simulink subsystem "Controls"  (R2024b)
settings: Solver=VariableStepAuto  StartTime=0.0  StopTime=10.0  RelTol=1e-3
undefined symbols (not defined in the file): D1, DiscIntNeverNeededParam, lag, Tctrl, test_alpha, Ts, Yg
libraries: powerlib_extras x74, simulink x10
(part 4 of 7)

== system Controls/Pole 1 Rectifier Control and Protection/Rectifier Controller/Voltage Error ==
  Vd_ref : Inport
  Vd_meas : Inport  Port=2
  Block : Inport  Port=3
  Id_err : Inport  Port=4
  Enable : EnablePort
  Constant1 : Constant  Value=0
  Constant2 : Constant  Value=0
  Constant3 : Constant  Value=Vd_marg
  Constant4 : Constant  Value=Id_marg
  Discrete 1st-Order Filter : powerlib_extras/Discrete  Control Blocks/Discrete 1st-Order Filter  FilterType=Highpass  Tc=0.01  Ts=dt  Initialize=off  Vac_Init=[0.8 -25 60]  Vdc_Init=-0.4  PlotResponse=off  param1=[1 500 0.1]
  MIN:eps MAX:inf : Saturate  UpperLimit=inf  LowerLimit=eps
  Math Function : Math  Operator=reciprocal  SignedPower=on
  Product1 : Product  Inputs=3  InputSameDT=on  SaturateOnIntegerOverflow=on  OutDataTypeStr=Inherit: Same as first input
  S6 : Subsystem  mask(Limiter with External Limits){}
      mask Display: disp('      Limiter\n')
  Sum3 : Sum  Inputs=+--  InputSameDT=on  SaturateOnIntegerOverflow=on  OutDataTypeStr=Inherit: Same as first input
  Switch2 : Switch  Threshold=0.5
  ERR_V : Outport
  wires:
  Sum3/1 -> Switch2/3
  Vd_ref/1 -> Sum3/1
  Vd_meas/1 -> Sum3/2
  Constant1/1 -> Switch2/1
  Block/1 -> Switch2/2
  Switch2/1 -> ERR_V/1  "ERR"
  Constant2/1 -> S6/3(MIN)
  S6/1("  ") -> Product1/3
  Math Function/1 -> Product1/2
  MIN:eps MAX:inf/1 -> Math Function/1
  Constant4/1 -> MIN:eps MAX:inf/1, S6/1(MAX)
  Product1/1 -> Discrete 1st-Order Filter/1
  Discrete 1st-Order Filter/1 -> Sum3/3  "dV"
  Id_err/1 -> S6/2(In)
  Constant3/1 -> Product1/1

== system Controls/Pole 1 Rectifier Control and Protection/Rectifier Controller/Voltage Regulator ==
  Max_i : Inport
  Min_i : Inport  Port=2
  ERR : Inport  Port=3
  Max_pi : Inport  Port=4
  Min_pi : Inport  Port=5
  Alpha_lin : Inport  Port=6
  Max_lin : Inport  Port=7
  Min_lin : Inport  Port=8
  Inv : Inport  Port=9
  Kp : Inport  Port=10
  Ki : Inport  Port=11
  Enable : EnablePort
  Voltage Regulator : Subsystem  mask(PI Regulator  With  External  Limits (Discrete)){Kp=Kp_V, Ki=Ki_V, IC_i=ICi_V, On_lin=on, pas=dt}
      mask prompts: Kp "Kp (deg/pu):"; Ki "Ki (deg/pu/s):"; IC_i "Integrator Initial Condition (deg):"; On_lin "Linearization  (On)"; pas "Sample time (s):"
      mask help: For the linearization it is important to specifie the mode of operation i.e. rectifier or inverter (negation of rectifier).
      mask Display: disp('PI Regulator\nWith external limits\n(Linearized Kp)\n(Discrete)\n\n')
  Alpha_ord : Outport
  wires:
  Kp/1 -> Voltage Regulator/10(Kp)
  Ki/1 -> Voltage Regulator/11(Ki)
  Voltage Regulator/1(Alpha_ord) -> Alpha_ord/1
  Max_i/1 -> Voltage Regulator/1(Max_i)
  Min_i/1 -> Voltage Regulator/2(Min_i)
  ERR/1 -> Voltage Regulator/3(ERR)
  Max_pi/1 -> Voltage Regulator/4(Max_pi)
  Min_pi/1 -> Voltage Regulator/5(Min_pi)
  Alpha_lin/1 -> Voltage Regulator/6(Alpha_lin)
  Max_lin/1 -> Voltage Regulator/7(Max_lin)
  Min_lin/1 -> Voltage Regulator/8(Min_lin)
  Inv/1 -> Voltage Regulator/9(Inv)

== system Controls/Pole 1 Rectifier Control and Protection/Rectifier Controller/alpha_init ==
  In1 : Inport  PortDimensions=1
  IC : InitialCondition  Value=min([ICi_V,ICi_I,ICi_G])
  Out1 : Outport
  wires:
  In1/1 -> IC/1
  IC/1 -> Out1/1

== system Controls/Pole 1 Rectifier Control and Protection/Rectifier Protections/DC Fault Protection (DCPROT) ==
  note: DC Fault Protection (only in Rectifier)
  VdL (pu) : Inport
  Deblocked : Inport  Port=2  OutDataTypeStr=boolean
  Lock : Inport  Port=3
  Enabled Subsystem : Subsystem  TreatAsAtomicUnit=on
  Forced_alpha : Outport
  wires:
  Enabled Subsystem/1(Forced_alpha) -> Forced_alpha/1
  Deblocked/1 -> Enabled Subsystem/2(Deblocked)
  Lock/1 -> Enabled Subsystem/3(Lock)
  VdL (pu)/1 -> Enabled Subsystem/1(VdL (pu))

== system Controls/Pole 1 Rectifier Control and Protection/Rectifier Protections/Informations ==
  note: The DC fault protection (DCPROT) and the Low AC voltage detection (LACVD) constitutes the
      | protectives functions at the rectifier. The DC fault protection detects a fault on the DC line and tries to
      | extinguish the fault current by ordering a Forced alpha operation during a fixed duration.
  note: DESCRIPTION
  note: Silvano Casoria (Hydro-Quebec)
  note: DC Protections - Rectifier
  note: The LACVD detects a low AC voltage condition on the rectifier commutation bus and sends a signal
      | (Lock) to the DCPROT in order to prevent the detection of a DC fault when the drop in the DC voltage is
      | due to a fault on the AC side. The LACVD at the inverter sends also a signal to lock the DCPROT for the
      | same reason.
  note: The  DCPROT detects a fault on the DC line and tries to extinguish the fault current by ordering a Forced
      | alpha operation for a fixed duration.

== system Controls/Pole 1 Rectifier Control and Protection/Rectifier Protections/Low AC Voltage Detection (LACVD) ==
  note: Low AC Voltage Detection
  Uac (pu) : Inport
  Enabled Subsystem : Subsystem  TreatAsAtomicUnit=on
  Low_AC_Voltage : Outport
  wires:
  Enabled Subsystem/1(Low_AC_Voltage) -> Low_AC_Voltage/1
  Uac (pu)/1 -> Enabled Subsystem/1(Uac (pu))

== system Controls/Pole 1 Rectifier Control and Protection/Rectifier Protections/Udio_6p ==
  note: Silvano Casoria
      | Power System Laboratory, IREQ
      | Hydro-Quebec
  note: Three-phase full-wave rectification
  Uabc (pu) : Inport
  MinMax : MinMax  Function=max  InputSameDT=on  SaturateOnIntegerOverflow=on
  MinMax1 : MinMax  InputSameDT=on  SaturateOnIntegerOverflow=on
  Sum : Sum  Inputs=+-  InputSameDT=on  SaturateOnIntegerOverflow=on  OutDataTypeStr=Inherit: Same as first input
  conversion pu ac->dc : Gain  Gain=pi/(3*sqrt(3))  SaturateOnIntegerOverflow=on  OutDataTypeStr=Inherit: Same as input  ParamDataTypeStr=Inherit: Same as input
  Udio_6p : Outport
  wires:
  MinMax1/1 -> Sum/2
  MinMax/1 -> Sum/1
  Uabc (pu)/1 -> MinMax/1, MinMax1/1
  Sum/1 -> conversion pu ac->dc/1
  conversion pu ac->dc/1 -> Udio_6p/1

== system Controls/Pole 2 Inverter Control and Protection/12-pulse Firing Control/PLL ==
  Vabc(pu) : Inport
  Constant : Constant  Value=2*pi/3
  Discrete 3-phase PLL : powerlib_extras/Discrete  Control Blocks/Discrete 3-phase PLL  Fmin=0.75 * PLL_f0  Par_Init="[PLL_ph  PLL_f0]"  ParK="[PLL_Kp  PLL_Ki]"  Ts=dt  AGC=off
  Sum : Sum  Inputs=|+-  SaturateOnIntegerOverflow=on
  Sum1 : Sum  Inputs=|++  SaturateOnIntegerOverflow=on
  Terminator : Terminator
  Trigonometric Function : Trigonometry
  Trigonometric Function1 : Trigonometry
  Trigonometric Function2 : Trigonometry
  Va : Outport
  Vb : Outport  Port=2
  Vc : Outport  Port=3
  Freq : Outport  Port=4
  wires:
  Discrete 3-phase PLL/3 -> Terminator/1
  Trigonometric Function2/1 -> Vc/1
  Trigonometric Function1/1 -> Vb/1
  Trigonometric Function/1 -> Va/1
  Sum1/1 -> Trigonometric Function2/1
  Constant/1 -> Sum/2, Sum1/2
  Sum/1 -> Trigonometric Function1/1
  Discrete 3-phase PLL/2 -> Sum1/1, Sum/1, Trigonometric Function/1
  Vabc(pu)/1 -> Discrete 3-phase PLL/1
  Discrete 3-phase PLL/1 -> Freq/1

== system Controls/Pole 2 Inverter Control and Protection/Inverter Current //Voltage//Gamma Controller /Alpha Control ==
  Forced_alpha : Inport
  D_alpha : Inport  Port=2
  Constant1 : Constant  Value=alpha_min
  Constant2 : Constant  Value=alpha_max
  Constant3 : Constant  Value=test_alpha
  Data Type Conversion : DataTypeConversion  OutDataTypeStr=boolean
  Logical Operator : Logic  Operator=OR
  "Rate Limiter " : RateLimiter  RisingSlewLimit=PRate_fix  FallingSlewLimit=NRate_fix  SampleTimeMode=inherited
  "Rate Limiter   " : RateLimiter  RisingSlewLimit=PRate_fix  FallingSlewLimit=NRate_fix  SampleTimeMode=inherited
  Sum : Sum  Inputs=-+  InputSameDT=on  SaturateOnIntegerOverflow=on  OutDataTypeStr=Inherit: Same as first input
  Switch : Switch  Threshold=0.5
  Switch1 : Switch  Threshold=0.5
  fixed alpha (deg) : Constant  Value=alpha_fix
  Max_i : Outport
  Min_i : Outport  Port=2
  wires:
  Data Type Conversion/1 -> Logical Operator/2
  Forced_alpha/1 -> Data Type Conversion/1
  fixed alpha (deg)/1 -> Switch1/1, Switch/1
  Switch1/1 -> "Rate Limiter   "/1
  Switch/1 -> "Rate Limiter "/1
  Constant1/1 -> Switch1/3
  Logical Operator/1 -> Switch1/2, Switch/2
  Constant3/1 -> Logical Operator/1
  Constant2/1 -> Sum/2
  Sum/1 -> Switch/3
  D_alpha/1 -> Sum/1
  "Rate Limiter "/1 -> Max_i/1
  "Rate Limiter   "/1 -> Min_i/1

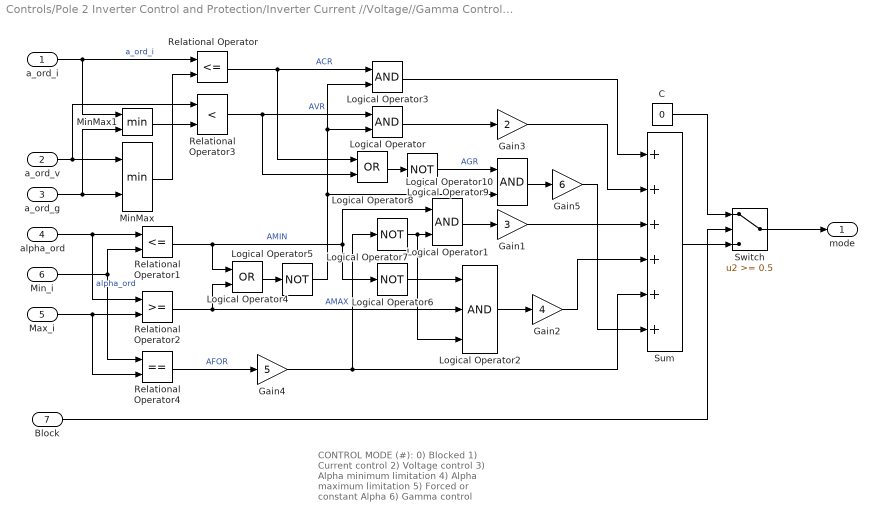
== system Controls/Pole 2 Inverter Control and Protection/Inverter Current //Voltage//Gamma Controller /Control Mode  ==
  note: CONTROL MODE (#):
      |
      | 0) Blocked
      | 1) Current control
      | 2) Voltage control
      | 3) Alpha minimum limitation
      | 4) Alpha maximum limitation
      | 5) Forced or constant Alpha
      | 6) Gamma control
  "a_ord_i " : Inport
  a_ord_v : Inport  Port=2
  a_ord_g : Inport  Port=3
  alpha_ord : Inport  Port=4
  Max_i : Inport  Port=5
  Min_i : Inport  Port=6
  Block : Inport  Port=7
  C : Constant  Value=0
  Gain1 : Gain  Gain=3  SaturateOnIntegerOverflow=on  OutDataTypeStr=Inherit: Same as input  ParamDataTypeStr=Inherit: Same as input
  Gain2 : Gain  Gain=4  SaturateOnIntegerOverflow=on  OutDataTypeStr=Inherit: Same as input  ParamDataTypeStr=Inherit: Same as input
  Gain3 : Gain  Gain=2  SaturateOnIntegerOverflow=on  OutDataTypeStr=Inherit: Same as input  ParamDataTypeStr=Inherit: Same as input
  Gain4 : Gain  Gain=5  SaturateOnIntegerOverflow=on  OutDataTypeStr=Inherit: Same as input  ParamDataTypeStr=Inherit: Same as input
  Gain5 : Gain  Gain=6  SaturateOnIntegerOverflow=on  OutDataTypeStr=Inherit: Same as input  ParamDataTypeStr=Inherit: Same as input
  Logical Operator{,1,3,10} (4 alike) : Logic
  Logical Operator2 : Logic  Inputs=3
  Logical Operator4 : Logic  Operator=OR
  Logical Operator{5..7,9} (4 alike) : Logic  Operator=NOT
  Logical Operator8 : Logic  Operator=OR
  MinMax : MinMax  Inputs=2  InputSameDT=on  SaturateOnIntegerOverflow=on
  MinMax1 : MinMax  Inputs=2  InputSameDT=on  SaturateOnIntegerOverflow=on
  Relational Operator : RelationalOperator  Operator=<=
  Relational Operator1 : RelationalOperator  Operator=<=
  Relational Operator2 : RelationalOperator
  Relational Operator3 : RelationalOperator  Operator=<
  Relational Operator4 : RelationalOperator  Operator===
  Sum : Sum  Inputs=++++++  InputSameDT=on  SaturateOnIntegerOverflow=on  OutDataTypeStr=Inherit: Same as first input
  Switch : Switch  Threshold=0.5
  mode : Outport
  wires:
  Logical Operator10/1 -> Gain5/1
  Logical Operator9/1 -> Logical Operator10/1  "AGR"
  MinMax1/1 -> Relational Operator3/2
  Gain5/1 -> Sum/6
  Logical Operator8/1 -> Logical Operator9/1
  MinMax/1 -> Relational Operator/2
  a_ord_g/1 -> MinMax1/2, MinMax/2
  a_ord_v/1 -> Relational Operator3/1, MinMax/1
  C/1 -> Switch/1
  Sum/1 -> Switch/3
  Switch/1 -> mode/1
  Block/1 -> Switch/2
  "a_ord_i "/1 -> MinMax1/1, Relational Operator/1  "a_ord_i"
  Relational Operator/1 -> Logical Operator8/1, Logical Operator3/1  "ACR"
  Logical Operator3/1 -> Sum/1
  Gain3/1 -> Sum/2
  Relational Operator3/1 -> Logical Operator8/2, Logical Operator/1  "AVR"
  Logical Operator/1 -> Gain3/1
  alpha_ord/1 -> Relational Operator1/1, Relational Operator2/1  "alpha_ord"
  Relational Operator1/1 -> Logical Operator4/1, Logical Operator6/1, Logical Operator1/1  "AMIN"
  Logical Operator4/1 -> Logical Operator5/1
  Relational Operator2/1 -> Logical Operator4/2, Logical Operator2/2  "AMAX"
  Logical Operator6/1 -> Logical Operator2/1
  Logical Operator2/1 -> Gain2/1
  Gain1/1 -> Sum/3
  Gain2/1 -> Sum/4
  Min_i/1 -> Relational Operator1/2, Relational Operator4/1
  Max_i/1 -> Relational Operator2/2, Relational Operator4/2
  Relational Operator4/1 -> Gain4/1  "AFOR"
  Logical Operator1/1 -> Gain1/1
  Gain4/1 -> Sum/5, Logical Operator7/1
  Logical Operator7/1 -> Logical Operator1/2, Logical Operator2/3
  Logical Operator5/1 -> Logical Operator10/2, Logical Operator/2, Logical Operator3/2

== system Controls/Pole 2 Inverter Control and Protection/Inverter Current //Voltage//Gamma Controller /Current Regulator ==
  note: PI Regulator With external limits (Linearized Kp) (Discrete)
  Max_i : Inport
  Min_i : Inport  Port=2
  ERR : Inport  Port=3
  Max_pi : Inport  Port=4
  Min_pi : Inport  Port=5
  Alpha_lin : Inport  Port=6
  Max_lin : Inport  Port=7
  Min_lin : Inport  Port=8
  Inv : Inport  Port=9
  Kp : Inport  Port=10
  Ki : Inport  Port=11
  Ground : Ground
  KI (deg per pu per s) : Gain  Gain=Ki  SaturateOnIntegerOverflow=on  OutDataTypeStr=Inherit: Same as input  ParamDataTypeStr=Inherit: Same as input
  Kp (deg per pu) : Constant  Value=Kp
  Kp Linearisation : Subsystem
  Prod : Product  InputSameDT=on  SaturateOnIntegerOverflow=on  OutDataTypeStr=Inherit: Same as first input
  Prod1 : Product  InputSameDT=on  SaturateOnIntegerOverflow=on  OutDataTypeStr=Inherit: Same as first input
  S16 : Subsystem  mask(Integrator  With  External  Dynamic  Limits (Discrete)){k=1, ic=IC_i, dt=dt}
      mask prompts: k "Gain:"; ic "Initial Condition:"; dt "Sample time: (s)"
      mask Display: disp('Integrator\nwith\nExternal Limits\nGain & Reset & Hold\n(Discrete)')
  S6 : Subsystem  mask(Limiter with External Limits){}
      mask Display: disp('      Limiter\n')
  Sum : Sum  InputSameDT=on  SaturateOnIntegerOverflow=on  OutDataTypeStr=Inherit: Same as first input
  Alpha_ord : Outport  InitialOutput=0
  wires:
  Prod1/1 -> S16/3(In)
  Ki/1 -> Prod1/2
  Kp/1 -> Kp Linearisation/2(Kp)
  Prod/1 -> Sum/1
  Min_lin/1 -> Kp Linearisation/4(Min_lin)
  Max_lin/1 -> Kp Linearisation/5(Max_lin)
  Inv/1 -> Kp Linearisation/3(Inv)
  Ground/1 -> S16/6(Reset Value), S16/5(Hold), S16/4(Reset)
  ERR/1 -> Prod1/1, Prod/2, KI (deg per pu per s)/1
  S16/1(Out) -> Sum/2
  Min_pi/1 -> S6/3(MIN)
  Max_pi/1 -> S6/1(MAX)
  Sum/1 -> S6/2(In)
  Min_i/1 -> S16/2(Min)
  Max_i/1 -> S16/1(Max)
  Kp Linearisation/1(Kp_lin) -> Prod/1
  S6/1("  ") -> Alpha_ord/1
  Alpha_lin/1 -> Kp Linearisation/1(Alpha_lin)

== system Controls/Pole 2 Inverter Control and Protection/Inverter Current //Voltage//Gamma Controller /Gamma Error ==
  G_ref : Inport
  G_meas : Inport  Port=2
  Block : Inport  Port=3
  Id_err : Inport  Port=4
  Enable : EnablePort
  Constant1 : Constant  Value=0
  Constant2 : Constant  Value=0
  Constant3 : Constant  Value=G_marg
  Constant4 : Constant  Value=Id_marg
  Discrete 1st-Order Filter : powerlib_extras/Discrete  Control Blocks/Discrete 1st-Order Filter  FilterType=Highpass  Tc=0.01  Ts=dt  Initialize=off  Vac_Init=[0.8 -25 60]  Vdc_Init=-0.4  PlotResponse=off  param1=[1 500 0.1]
  MIN:eps MAX:inf : Saturate  UpperLimit=inf  LowerLimit=eps
  Math Function : Math  Operator=reciprocal  SignedPower=on
  Product1 : Product  Inputs=3  InputSameDT=on  SaturateOnIntegerOverflow=on  OutDataTypeStr=Inherit: Same as first input
  S6 : Subsystem  mask(Limiter with External Limits){}
      mask Display: disp('      Limiter\n')
  Sum3 : Sum  Inputs=-+-  InputSameDT=on  SaturateOnIntegerOverflow=on  OutDataTypeStr=Inherit: Same as first input
  Switch2 : Switch  Threshold=0.5
  ERR_G : Outport
  wires:
  Constant3/1 -> Product1/1
  Id_err/1 -> S6/2(In)
  Discrete 1st-Order Filter/1 -> Sum3/3  "dG"
  Product1/1 -> Discrete 1st-Order Filter/1
  Constant4/1 -> S6/1(MAX), MIN:eps MAX:inf/1
  MIN:eps MAX:inf/1 -> Math Function/1
  Math Function/1 -> Product1/2
  S6/1("  ") -> Product1/3
  Constant2/1 -> S6/3(MIN)
  Switch2/1 -> ERR_G/1  "ERR"
  Block/1 -> Switch2/2
  Constant1/1 -> Switch2/1
  G_meas/1 -> Sum3/2
  G_ref/1 -> Sum3/1
  Sum3/1 -> Switch2/3

== system Controls/Pole 2 Inverter Control and Protection/Inverter Current //Voltage//Gamma Controller /Gamma Regulator ==
  Max_i : Inport
  Min_i : Inport  Port=2
  ERR : Inport  Port=3
  Max_pi : Inport  Port=4
  Min_pi : Inport  Port=5
  Alpha_lin : Inport  Port=6
  Max_lin : Inport  Port=7
  Min_lin : Inport  Port=8
  Inv : Inport  Port=9
  Kp : Inport  Port=10
  Ki : Inport  Port=11
  Enable : EnablePort
  Gamma Regulator : Subsystem  mask(PI Regulator  With  External  Limits (Discrete)){Kp=Kp_G, Ki=Ki_G, IC_i=ICi_G, On_lin=on, pas=dt}
      mask prompts: Kp "Kp (deg/pu):"; Ki "Ki (deg/pu/s):"; IC_i "Integrator Initial Condition (deg):"; On_lin "Linearization  (On)"; pas "Sample time (s):"
      mask help: For the linearization it is important to specifie the mode of operation i.e. rectifier or inverter (negation of rectifier).
      mask Display: disp('PI Regulator\nWith external limits\n(Linearized Kp)\n(Discrete)\n\n')
  Alpha_ord : Outport
  wires:
  Ki/1 -> Gamma Regulator/11(Ki)
  Kp/1 -> Gamma Regulator/10(Kp)
  Inv/1 -> Gamma Regulator/9(Inv)
  Min_lin/1 -> Gamma Regulator/8(Min_lin)
  Max_lin/1 -> Gamma Regulator/7(Max_lin)
  Alpha_lin/1 -> Gamma Regulator/6(Alpha_lin)
  Min_pi/1 -> Gamma Regulator/5(Min_pi)
  Max_pi/1 -> Gamma Regulator/4(Max_pi)
  ERR/1 -> Gamma Regulator/3(ERR)
  Min_i/1 -> Gamma Regulator/2(Min_i)
  Max_i/1 -> Gamma Regulator/1(Max_i)
  Gamma Regulator/1(Alpha_ord) -> Alpha_ord/1

== system Controls/Pole 2 Inverter Control and Protection/Inverter Current //Voltage//Gamma Controller /Voltage Dependant Current Order Limiter ==
  note: Voltage Dependant Current Order Limiter (VDCOL) (Discrete)
  Id_ref (pu) : Inport
  Vd (pu) : Inport  Port=2
  Constant : Constant  Value=Id_min
  Constant1 : Constant  Value=Vd_min
  Constant2 : Constant  Value=Vd_seuil
  Constant3 : Constant
  Constant4 : Constant
  Constant5 : Constant  Value=Tu
  Logical Operator : Logic  Operator=NOT
  Math Function : Math  Operator=reciprocal  SignedPower=on
  Max = 10 Min=Id_min_abs : Saturate  UpperLimit=10  LowerLimit=Id_min_abs
  MinMax2 : MinMax  Function=max  Inputs=2  InputSameDT=on  SaturateOnIntegerOverflow=on
  MinMax3 : MinMax  Inputs=2  InputSameDT=on  SaturateOnIntegerOverflow=on
  PB_R : Subsystem  mask(Low Pass Filter With Reset (discrete: Zoh method, Forward Euler)){ic=1, dt=pas}
      mask prompts: ic "Initial condition:"; dt "Sample time (s)"
      mask help:
      | The output will be reset to the input value (Time constant = 0)  during the input (2) is True. The Time constant (T) is defined by
      | input (3).
      mask Display:
      | plot(0,0,100,100,[90,80,70,60,50,40,29,20,10],[60,55,52,55,60,65,67,65,60],[89,80,71,60,50,40,30,20,10],[40,35,32,35,40,45,47,45,40],[56,44],[70,50]);
      | disp('\n\nD')
  Product : Product  InputSameDT=on  SaturateOnIntegerOverflow=on
  Product1 : Product  InputSameDT=on  SaturateOnIntegerOverflow=on
  Product2 : Product  InputSameDT=on  SaturateOnIntegerOverflow=on  OutDataTypeStr=Inherit: Same as first input
  Product3 : Product  InputSameDT=on  SaturateOnIntegerOverflow=on  OutDataTypeStr=Inherit: Same as first input
  Product4 : Product  InputSameDT=on  SaturateOnIntegerOverflow=on  OutDataTypeStr=Inherit: Same as first input
  Relational Operator : RelationalOperator
  Sum : Sum  Inputs=+-  InputSameDT=on  SaturateOnIntegerOverflow=on  OutDataTypeStr=Inherit: Same as first input
  Sum1 : Sum  Inputs=+-  InputSameDT=on  SaturateOnIntegerOverflow=on  OutDataTypeStr=Inherit: Same as first input
  Sum2 : Sum  Inputs=+-  InputSameDT=on  SaturateOnIntegerOverflow=on  OutDataTypeStr=Inherit: Same as first input
  Sum3 : Sum  InputSameDT=on  SaturateOnIntegerOverflow=on  OutDataTypeStr=Inherit: Same as first input
  Unit Delay : UnitDelay  SampleTime=pas  HasFrameUpgradeWarning=on
  Id_ref_lim : Outport  InitialOutput=0
  Vd_filt : Outport  Port=2  InitialOutput=0
  wires:
  Logical Operator/1 -> PB_R/2(Reset)
  Unit Delay/1 -> Logical Operator/1
  Vd (pu)/1 -> Relational Operator/1, PB_R/1("In ")
  PB_R/1(Out) -> Relational Operator/2, Vd_filt/1, Product2/2
  Constant5/1 -> PB_R/3(T)
  Constant3/1 -> Sum/1
  Constant1/1 -> Sum1/2
  Sum1/1 -> Math Function/1
  Sum/1 -> Product/1
  Math Function/1 -> Product/2
  Constant4/1 -> Sum2/1
  Sum2/1 -> Sum3/1  "B"
  Product2/1 -> Sum3/2
  Sum3/1 -> Product1/2
  Constant/1 -> Sum/2, Product4/1
  Product4/1 -> Max = 10 Min=Id_min_abs/1  "min"
  Id_ref (pu)/1 -> Product1/1, MinMax3/1, Product4/2
  MinMax3/1 -> Id_ref_lim/1
  Product3/1 -> Sum2/2
  Product/1 -> Product2/1, Product3/2  "A"
  Constant2/1 -> Sum1/1, Product3/1
  Product1/1 -> MinMax2/1  "Idref_lim"
  MinMax2/1 -> MinMax3/2
  Max = 10 Min=Id_min_abs/1 -> MinMax2/2
  Relational Operator/1 -> Unit Delay/1

== system Controls/Pole 2 Inverter Control and Protection/Inverter Current //Voltage//Gamma Controller /Voltage Error ==
  Vd_ref : Inport
  Vd_meas : Inport  Port=2
  Block : Inport  Port=3
  Id_err : Inport  Port=4
  Enable : EnablePort
  Constant1 : Constant  Value=0
  Constant2 : Constant  Value=0
  Constant3 : Constant  Value=Vd_marg
  Constant4 : Constant  Value=Id_marg
  Discrete 1st-Order Filter : powerlib_extras/Discrete  Control Blocks/Discrete 1st-Order Filter  FilterType=Highpass  Tc=0.01  Ts=dt  Initialize=off  Vac_Init=[0.8 -25 60]  Vdc_Init=-0.4  PlotResponse=off  param1=[1 500 0.1]
  MIN:eps MAX:inf : Saturate  UpperLimit=inf  LowerLimit=eps
  Math Function : Math  Operator=reciprocal  SignedPower=on
  Product1 : Product  Inputs=3  InputSameDT=on  SaturateOnIntegerOverflow=on  OutDataTypeStr=Inherit: Same as first input
  S6 : Subsystem  mask(Limiter with External Limits){}
      mask Display: disp('      Limiter\n')
  Sum3 : Sum  Inputs=+--  InputSameDT=on  SaturateOnIntegerOverflow=on  OutDataTypeStr=Inherit: Same as first input
  Switch2 : Switch  Threshold=0.5
  ERR_V : Outport
  wires:
  Sum3/1 -> Switch2/3
  Vd_ref/1 -> Sum3/1
  Vd_meas/1 -> Sum3/2
  Constant1/1 -> Switch2/1
  Block/1 -> Switch2/2
  Switch2/1 -> ERR_V/1  "ERR"
  Constant2/1 -> S6/3(MIN)
  S6/1("  ") -> Product1/3
  Math Function/1 -> Product1/2
  MIN:eps MAX:inf/1 -> Math Function/1
  Constant4/1 -> MIN:eps MAX:inf/1, S6/1(MAX)
  Product1/1 -> Discrete 1st-Order Filter/1
  Discrete 1st-Order Filter/1 -> Sum3/3  "dV"
  Id_err/1 -> S6/2(In)
  Constant3/1 -> Product1/1

== system Controls/Pole 2 Inverter Control and Protection/Inverter Current //Voltage//Gamma Controller /Voltage Regulator ==
  Max_i : Inport
  Min_i : Inport  Port=2
  ERR : Inport  Port=3
  Max_pi : Inport  Port=4
  Min_pi : Inport  Port=5
  Alpha_lin : Inport  Port=6
  Max_lin : Inport  Port=7
  Min_lin : Inport  Port=8
  Inv : Inport  Port=9
  Kp : Inport  Port=10
  Ki : Inport  Port=11
  Enable : EnablePort
  Voltage Regulator : Subsystem  mask(PI Regulator  With  External  Limits (Discrete)){Kp=Kp_V, Ki=Ki_V, IC_i=ICi_V, On_lin=on, pas=dt}
      mask prompts: Kp "Kp (deg/pu):"; Ki "Ki (deg/pu/s):"; IC_i "Integrator Initial Condition (deg):"; On_lin "Linearization  (On)"; pas "Sample time (s):"
      mask help: For the linearization it is important to specifie the mode of operation i.e. rectifier or inverter (negation of rectifier).
      mask Display: disp('PI Regulator\nWith external limits\n(Linearized Kp)\n(Discrete)\n\n')
  Alpha_ord : Outport
  wires:
  Ki/1 -> Voltage Regulator/11(Ki)
  Kp/1 -> Voltage Regulator/10(Kp)
  Voltage Regulator/1(Alpha_ord) -> Alpha_ord/1
  Max_i/1 -> Voltage Regulator/1(Max_i)
  Min_i/1 -> Voltage Regulator/2(Min_i)
  ERR/1 -> Voltage Regulator/3(ERR)
  Max_pi/1 -> Voltage Regulator/4(Max_pi)
  Min_pi/1 -> Voltage Regulator/5(Min_pi)
  Alpha_lin/1 -> Voltage Regulator/6(Alpha_lin)
  Max_lin/1 -> Voltage Regulator/7(Max_lin)
  Min_lin/1 -> Voltage Regulator/8(Min_lin)
  Inv/1 -> Voltage Regulator/9(Inv)

== system Controls/Pole 2 Inverter Control and Protection/Inverter Current //Voltage//Gamma Controller /alpha_init ==
  In1 : Inport  PortDimensions=1
  IC : InitialCondition  Value=min([ICi_V,ICi_I,ICi_G])
  Out1 : Outport
  wires:
  In1/1 -> IC/1
  IC/1 -> Out1/1

== system Controls/Pole 2 Inverter Control and Protection/Inverter Protections/Commutation Failure Prevention Control (CFPREV) ==
  note: Commutation failure Prevention Control Module (CFPREV)
  Uabc (pu) : Inport
  C : Constant  Value=STATE
  Enabled Subsystem : Subsystem  TreatAsAtomicUnit=on
  AMIN_CFPREV (deg) : Outport
  wires:
  Enabled Subsystem/1(AMIN_CFPREV (deg)) -> AMIN_CFPREV (deg)/1
  Uabc (pu)/1 -> Enabled Subsystem/1(Uabc (pu))
  C/1 -> Enabled Subsystem/Enable

== system Controls/Pole 2 Inverter Control and Protection/Inverter Protections/Informations ==
  note: NOTE 1: Result of a failure of the incoming valve to take over the direct current before the commutating voltage reverses its polarity.
  note: DC Protections - Inverter
  note: DESCRIPTION
  note: The LACVD detects a low AC voltage condition on the inverter commutation bus and sends a signal
      | (Lock) to the DCPROT (in the rectifier) in order to prevent the detection of a DC fault when the drop in
      | the DC voltage is due to a fault on the AC side. The LACVD at the irectifier sends also a signal to
      | lock the DCPROT for the same reason.
  note: The Commutation failure prevention control (CFPREV) and the Low AC voltage detection (LACVD)
      | constitutes the protective functions at the rinverter.
  note: The CFPREV  mitigates commutation failures due to AC voltage dips. After a fault detection (three-phase or
      | one-phase) an angle value (AMIN_CFPREV) is sent to the converter control in order to be deducted from the
      | maximum delay angle limit (alpha_max). In practice, the commutation margin is consequently enlarged
      | reducing therefore the risk of commutation failures (note 1).

== system Controls/Pole 2 Inverter Control and Protection/Inverter Protections/Low AC Voltage Detection (LACVD) ==
  note: Low AC Voltage Detection
  Uac (pu) : Inport
  Enabled Subsystem : Subsystem  TreatAsAtomicUnit=on
  Low_AC_Voltage : Outport
  wires:
  Enabled Subsystem/1(Low_AC_Voltage) -> Low_AC_Voltage/1
  Uac (pu)/1 -> Enabled Subsystem/1(Uac (pu))

== system Controls/Pole 2 Inverter Control and Protection/Inverter Protections/Udio_6p ==
  note: Three-phase full-wave rectification
  note: Silvano Casoria
      | Power System Laboratory, IREQ
      | Hydro-Quebec
  Uabc (pu) : Inport
  MinMax : MinMax  Function=max  InputSameDT=on  SaturateOnIntegerOverflow=on
  MinMax1 : MinMax  InputSameDT=on  SaturateOnIntegerOverflow=on
  Sum : Sum  Inputs=+-  InputSameDT=on  SaturateOnIntegerOverflow=on  OutDataTypeStr=Inherit: Same as first input
  conversion pu ac->dc : Gain  Gain=pi/(3*sqrt(3))  SaturateOnIntegerOverflow=on  OutDataTypeStr=Inherit: Same as input  ParamDataTypeStr=Inherit: Same as input
  Udio_6p : Outport
  wires:
  conversion pu ac->dc/1 -> Udio_6p/1
  Sum/1 -> conversion pu ac->dc/1
  Uabc (pu)/1 -> MinMax1/1, MinMax/1
  MinMax/1 -> Sum/1
  MinMax1/1 -> Sum/2

== system Controls/Pole 2 Rectifier Control and Protection/12-pulse Firing Control/PLL ==
  Vabc(pu) : Inport
  Constant : Constant  Value=2*pi/3
  Discrete 3-phase PLL : powerlib_extras/Discrete  Control Blocks/Discrete 3-phase PLL  Fmin=0.75 * PLL_f0  Par_Init="[PLL_ph  PLL_f0]"  ParK="[PLL_Kp  PLL_Ki]"  Ts=dt  AGC=off
  Sum : Sum  Inputs=|+-  SaturateOnIntegerOverflow=on
  Sum1 : Sum  Inputs=|++  SaturateOnIntegerOverflow=on
  Terminator : Terminator
  Trigonometric Function : Trigonometry
  Trigonometric Function1 : Trigonometry
  Trigonometric Function2 : Trigonometry
  Va : Outport
  Vb : Outport  Port=2
  Vc : Outport  Port=3
  Freq : Outport  Port=4
  wires:
  Discrete 3-phase PLL/3 -> Terminator/1
  Trigonometric Function2/1 -> Vc/1
  Trigonometric Function1/1 -> Vb/1
  Trigonometric Function/1 -> Va/1
  Sum1/1 -> Trigonometric Function2/1
  Constant/1 -> Sum/2, Sum1/2
  Sum/1 -> Trigonometric Function1/1
  Discrete 3-phase PLL/2 -> Sum1/1, Sum/1, Trigonometric Function/1
  Vabc(pu)/1 -> Discrete 3-phase PLL/1
  Discrete 3-phase PLL/1 -> Freq/1

== system Controls/Pole 2 Rectifier Control and Protection/Rectifier Controller/Alpha Control ==
  Forced_alpha : Inport
  D_alpha : Inport  Port=2
  Constant1 : Constant  Value=alpha_min
  Constant2 : Constant  Value=alpha_max
  Constant3 : Constant  Value=test_alpha
  Data Type Conversion : DataTypeConversion  OutDataTypeStr=boolean
  Logical Operator : Logic  Operator=OR
  "Rate Limiter " : RateLimiter  RisingSlewLimit=PRate_fix  FallingSlewLimit=NRate_fix  SampleTimeMode=inherited
  "Rate Limiter   " : RateLimiter  RisingSlewLimit=PRate_fix  FallingSlewLimit=NRate_fix  SampleTimeMode=inherited
  Sum : Sum  Inputs=-+  InputSameDT=on  SaturateOnIntegerOverflow=on  OutDataTypeStr=Inherit: Same as first input
  Switch : Switch  Threshold=0.5
  Switch1 : Switch  Threshold=0.5
  fixed alpha (deg) : Constant  Value=alpha_fix
  Max_i : Outport
  Min_i : Outport  Port=2
  wires:
  Data Type Conversion/1 -> Logical Operator/2
  Forced_alpha/1 -> Data Type Conversion/1
  fixed alpha (deg)/1 -> Switch1/1, Switch/1
  Switch1/1 -> "Rate Limiter   "/1
  Switch/1 -> "Rate Limiter "/1
  Constant1/1 -> Switch1/3
  Logical Operator/1 -> Switch1/2, Switch/2
  Constant3/1 -> Logical Operator/1
  Constant2/1 -> Sum/2
  Sum/1 -> Switch/3
  D_alpha/1 -> Sum/1
  "Rate Limiter "/1 -> Max_i/1
  "Rate Limiter   "/1 -> Min_i/1

== system Controls/Pole 2 Rectifier Control and Protection/Rectifier Controller/Control Mode  ==
  note: CONTROL MODE (#):
      |
      | 0) Blocked
      | 1) Current control
      | 2) Voltage control
      | 3) Alpha minimum limitation
      | 4) Alpha maximum limitation
      | 5) Forced or constant Alpha
      | 6) Gamma control
  "a_ord_i " : Inport
  a_ord_v : Inport  Port=2
  a_ord_g : Inport  Port=3
  alpha_ord : Inport  Port=4
  Max_i : Inport  Port=5
  Min_i : Inport  Port=6
  Block : Inport  Port=7
  C : Constant  Value=0
  Gain1 : Gain  Gain=3  SaturateOnIntegerOverflow=on  OutDataTypeStr=Inherit: Same as input  ParamDataTypeStr=Inherit: Same as input
  Gain2 : Gain  Gain=4  SaturateOnIntegerOverflow=on  OutDataTypeStr=Inherit: Same as input  ParamDataTypeStr=Inherit: Same as input
  Gain3 : Gain  Gain=2  SaturateOnIntegerOverflow=on  OutDataTypeStr=Inherit: Same as input  ParamDataTypeStr=Inherit: Same as input
  Gain4 : Gain  Gain=5  SaturateOnIntegerOverflow=on  OutDataTypeStr=Inherit: Same as input  ParamDataTypeStr=Inherit: Same as input
  Gain5 : Gain  Gain=6  SaturateOnIntegerOverflow=on  OutDataTypeStr=Inherit: Same as input  ParamDataTypeStr=Inherit: Same as input
  Logical Operator{,1,3,10} (4 alike) : Logic
  Logical Operator2 : Logic  Inputs=3
  Logical Operator4 : Logic  Operator=OR
  Logical Operator{5..7,9} (4 alike) : Logic  Operator=NOT
  Logical Operator8 : Logic  Operator=OR
  MinMax : MinMax  Inputs=2  InputSameDT=on  SaturateOnIntegerOverflow=on
  MinMax1 : MinMax  Inputs=2  InputSameDT=on  SaturateOnIntegerOverflow=on
  Relational Operator : RelationalOperator  Operator=<=
  Relational Operator1 : RelationalOperator  Operator=<=
  Relational Operator2 : RelationalOperator
  Relational Operator3 : RelationalOperator  Operator=<
  Relational Operator4 : RelationalOperator  Operator===
  Sum : Sum  Inputs=++++++  InputSameDT=on  SaturateOnIntegerOverflow=on  OutDataTypeStr=Inherit: Same as first input
  Switch : Switch  Threshold=0.5
  mode : Outport
  wires:
  Logical Operator10/1 -> Gain5/1
  Logical Operator9/1 -> Logical Operator10/1  "AGR"
  MinMax1/1 -> Relational Operator3/2
  Gain5/1 -> Sum/6
  Logical Operator8/1 -> Logical Operator9/1
  MinMax/1 -> Relational Operator/2
  a_ord_g/1 -> MinMax1/2, MinMax/2
  a_ord_v/1 -> Relational Operator3/1, MinMax/1
  C/1 -> Switch/1
  Sum/1 -> Switch/3
  Switch/1 -> mode/1
  Block/1 -> Switch/2
  "a_ord_i "/1 -> MinMax1/1, Relational Operator/1  "a_ord_i"
  Relational Operator/1 -> Logical Operator8/1, Logical Operator3/1  "ACR"
  Logical Operator3/1 -> Sum/1
  Gain3/1 -> Sum/2
  Relational Operator3/1 -> Logical Operator8/2, Logical Operator/1  "AVR"
  Logical Operator/1 -> Gain3/1
  alpha_ord/1 -> Relational Operator1/1, Relational Operator2/1  "alpha_ord"
  Relational Operator1/1 -> Logical Operator4/1, Logical Operator6/1, Logical Operator1/1  "AMIN"
  Logical Operator4/1 -> Logical Operator5/1
  Relational Operator2/1 -> Logical Operator4/2, Logical Operator2/2  "AMAX"
  Logical Operator6/1 -> Logical Operator2/1
  Logical Operator2/1 -> Gain2/1
  Gain1/1 -> Sum/3
  Gain2/1 -> Sum/4
  Min_i/1 -> Relational Operator1/2, Relational Operator4/1
  Max_i/1 -> Relational Operator2/2, Relational Operator4/2
  Relational Operator4/1 -> Gain4/1  "AFOR"
  Logical Operator1/1 -> Gain1/1
  Gain4/1 -> Sum/5, Logical Operator7/1
  Logical Operator7/1 -> Logical Operator1/2, Logical Operator2/3
  Logical Operator5/1 -> Logical Operator10/2, Logical Operator/2, Logical Operator3/2

== system Controls/Pole 2 Rectifier Control and Protection/Rectifier Controller/Current Regulator ==
  note: PI Regulator With external limits (Linearized Kp) (Discrete)
  Max_i : Inport
  Min_i : Inport  Port=2
  ERR : Inport  Port=3
  Max_pi : Inport  Port=4
  Min_pi : Inport  Port=5
  Alpha_lin : Inport  Port=6
  Max_lin : Inport  Port=7
  Min_lin : Inport  Port=8
  Inv : Inport  Port=9
  Kp : Inport  Port=10
  Ki : Inport  Port=11
  Ground : Ground
  KI (deg per pu per s) : Gain  Gain=Ki  SaturateOnIntegerOverflow=on  OutDataTypeStr=Inherit: Same as input  ParamDataTypeStr=Inherit: Same as input
  Kp (deg per pu) : Constant  Value=Kp
  Kp Linearisation : Subsystem
  Prod : Product  InputSameDT=on  SaturateOnIntegerOverflow=on  OutDataTypeStr=Inherit: Same as first input
  Prod1 : Product  InputSameDT=on  SaturateOnIntegerOverflow=on  OutDataTypeStr=Inherit: Same as first input
  S16 : Subsystem  mask(Integrator  With  External  Dynamic  Limits (Discrete)){k=1, ic=IC_i, dt=dt}
      mask prompts: k "Gain:"; ic "Initial Condition:"; dt "Sample time: (s)"
      mask Display: disp('Integrator\nwith\nExternal Limits\nGain & Reset & Hold\n(Discrete)')
  S6 : Subsystem  mask(Limiter with External Limits){}
      mask Display: disp('      Limiter\n')
  Sum : Sum  InputSameDT=on  SaturateOnIntegerOverflow=on  OutDataTypeStr=Inherit: Same as first input
  Alpha_ord : Outport  InitialOutput=0
  wires:
  Prod1/1 -> S16/3(In)
  Ki/1 -> Prod1/2
  Kp/1 -> Kp Linearisation/2(Kp)
  Prod/1 -> Sum/1
  Min_lin/1 -> Kp Linearisation/4(Min_lin)
  Max_lin/1 -> Kp Linearisation/5(Max_lin)
  Inv/1 -> Kp Linearisation/3(Inv)
  Ground/1 -> S16/6(Reset Value), S16/5(Hold), S16/4(Reset)
  ERR/1 -> Prod1/1, Prod/2, KI (deg per pu per s)/1
  S16/1(Out) -> Sum/2
  Min_pi/1 -> S6/3(MIN)
  Max_pi/1 -> S6/1(MAX)
  Sum/1 -> S6/2(In)
  Min_i/1 -> S16/2(Min)
  Max_i/1 -> S16/1(Max)
  Kp Linearisation/1(Kp_lin) -> Prod/1
  S6/1("  ") -> Alpha_ord/1
  Alpha_lin/1 -> Kp Linearisation/1(Alpha_lin)

== system Controls/Pole 2 Rectifier Control and Protection/Rectifier Controller/Gamma Error ==
  G_ref : Inport
  G_meas : Inport  Port=2
  Block : Inport  Port=3
  Id_err : Inport  Port=4
  Enable : EnablePort
  Constant1 : Constant  Value=0
  Constant2 : Constant  Value=0
  Constant3 : Constant  Value=G_marg
  Constant4 : Constant  Value=Id_marg
  Discrete 1st-Order Filter : powerlib_extras/Discrete  Control Blocks/Discrete 1st-Order Filter  FilterType=Highpass  Tc=0.01  Ts=dt  Initialize=off  Vac_Init=[0.8 -25 60]  Vdc_Init=-0.4  PlotResponse=off  param1=[1 500 0.1]
  MIN:eps MAX:inf : Saturate  UpperLimit=inf  LowerLimit=eps
  Math Function : Math  Operator=reciprocal  SignedPower=on
  Product1 : Product  Inputs=3  InputSameDT=on  SaturateOnIntegerOverflow=on  OutDataTypeStr=Inherit: Same as first input
  S6 : Subsystem  mask(Limiter with External Limits){}
      mask Display: disp('      Limiter\n')
  Sum3 : Sum  Inputs=-+-  InputSameDT=on  SaturateOnIntegerOverflow=on  OutDataTypeStr=Inherit: Same as first input
  Switch2 : Switch  Threshold=0.5
  ERR_G : Outport
  wires:
  Constant3/1 -> Product1/1
  Id_err/1 -> S6/2(In)
  Discrete 1st-Order Filter/1 -> Sum3/3  "dG"
  Product1/1 -> Discrete 1st-Order Filter/1
  Constant4/1 -> S6/1(MAX), MIN:eps MAX:inf/1
  MIN:eps MAX:inf/1 -> Math Function/1
  Math Function/1 -> Product1/2
  S6/1("  ") -> Product1/3
  Constant2/1 -> S6/3(MIN)
  Switch2/1 -> ERR_G/1  "ERR"
  Block/1 -> Switch2/2
  Constant1/1 -> Switch2/1
  G_meas/1 -> Sum3/2
  G_ref/1 -> Sum3/1
  Sum3/1 -> Switch2/3

== system Controls/Pole 2 Rectifier Control and Protection/Rectifier Controller/Gamma Regulator ==
  Max_i : Inport
  Min_i : Inport  Port=2
  ERR : Inport  Port=3
  Max_pi : Inport  Port=4
  Min_pi : Inport  Port=5
  Alpha_lin : Inport  Port=6
  Max_lin : Inport  Port=7
  Min_lin : Inport  Port=8
  Inv : Inport  Port=9
  Kp : Inport  Port=10
  Ki : Inport  Port=11
  Enable : EnablePort
  Gamma Regulator : Subsystem  mask(PI Regulator  With  External  Limits (Discrete)){Kp=Kp_G, Ki=Ki_G, IC_i=ICi_G, On_lin=on, pas=dt}
      mask prompts: Kp "Kp (deg/pu):"; Ki "Ki (deg/pu/s):"; IC_i "Integrator Initial Condition (deg):"; On_lin "Linearization  (On)"; pas "Sample time (s):"
      mask help: For the linearization it is important to specifie the mode of operation i.e. rectifier or inverter (negation of rectifier).
      mask Display: disp('PI Regulator\nWith external limits\n(Linearized Kp)\n(Discrete)\n\n')
  Alpha_ord : Outport
  wires:
  Ki/1 -> Gamma Regulator/11(Ki)
  Kp/1 -> Gamma Regulator/10(Kp)
  Inv/1 -> Gamma Regulator/9(Inv)
  Min_lin/1 -> Gamma Regulator/8(Min_lin)
  Max_lin/1 -> Gamma Regulator/7(Max_lin)
  Alpha_lin/1 -> Gamma Regulator/6(Alpha_lin)
  Min_pi/1 -> Gamma Regulator/5(Min_pi)
  Max_pi/1 -> Gamma Regulator/4(Max_pi)
  ERR/1 -> Gamma Regulator/3(ERR)
  Min_i/1 -> Gamma Regulator/2(Min_i)
  Max_i/1 -> Gamma Regulator/1(Max_i)
  Gamma Regulator/1(Alpha_ord) -> Alpha_ord/1

== system Controls/Pole 2 Rectifier Control and Protection/Rectifier Controller/Voltage Dependant Current Order Limiter ==
  note: Voltage Dependant Current Order Limiter (VDCOL) (Discrete)
  Id_ref (pu) : Inport
  Vd (pu) : Inport  Port=2
  Constant : Constant  Value=Id_min
  Constant1 : Constant  Value=Vd_min
  Constant2 : Constant  Value=Vd_seuil
  Constant3 : Constant
  Constant4 : Constant
  Constant5 : Constant  Value=Tu
  Logical Operator : Logic  Operator=NOT
  Math Function : Math  Operator=reciprocal  SignedPower=on
  Max = 10 Min=Id_min_abs : Saturate  UpperLimit=10  LowerLimit=Id_min_abs
  MinMax2 : MinMax  Function=max  Inputs=2  InputSameDT=on  SaturateOnIntegerOverflow=on
  MinMax3 : MinMax  Inputs=2  InputSameDT=on  SaturateOnIntegerOverflow=on
  PB_R : Subsystem  mask(Low Pass Filter With Reset (discrete: Zoh method, Forward Euler)){ic=1, dt=pas}
      mask prompts: ic "Initial condition:"; dt "Sample time (s)"
      mask help:
      | The output will be reset to the input value (Time constant = 0)  during the input (2) is True. The Time constant (T) is defined by
      | input (3).
      mask Display:
      | plot(0,0,100,100,[90,80,70,60,50,40,29,20,10],[60,55,52,55,60,65,67,65,60],[89,80,71,60,50,40,30,20,10],[40,35,32,35,40,45,47,45,40],[56,44],[70,50]);
      | disp('\n\nD')
  Product : Product  InputSameDT=on  SaturateOnIntegerOverflow=on
  Product1 : Product  InputSameDT=on  SaturateOnIntegerOverflow=on
  Product2 : Product  InputSameDT=on  SaturateOnIntegerOverflow=on  OutDataTypeStr=Inherit: Same as first input
  Product3 : Product  InputSameDT=on  SaturateOnIntegerOverflow=on  OutDataTypeStr=Inherit: Same as first input
  Product4 : Product  InputSameDT=on  SaturateOnIntegerOverflow=on  OutDataTypeStr=Inherit: Same as first input
  Relational Operator : RelationalOperator
  Sum : Sum  Inputs=+-  InputSameDT=on  SaturateOnIntegerOverflow=on  OutDataTypeStr=Inherit: Same as first input
  Sum1 : Sum  Inputs=+-  InputSameDT=on  SaturateOnIntegerOverflow=on  OutDataTypeStr=Inherit: Same as first input
  Sum2 : Sum  Inputs=+-  InputSameDT=on  SaturateOnIntegerOverflow=on  OutDataTypeStr=Inherit: Same as first input
  Sum3 : Sum  InputSameDT=on  SaturateOnIntegerOverflow=on  OutDataTypeStr=Inherit: Same as first input
  Unit Delay : UnitDelay  SampleTime=pas  HasFrameUpgradeWarning=on
  Id_ref_lim : Outport  InitialOutput=0
  Vd_filt : Outport  Port=2  InitialOutput=0
  wires:
  Logical Operator/1 -> PB_R/2(Reset)
  Unit Delay/1 -> Logical Operator/1
  Vd (pu)/1 -> Relational Operator/1, PB_R/1("In ")
  PB_R/1(Out) -> Relational Operator/2, Vd_filt/1, Product2/2
  Constant5/1 -> PB_R/3(T)
  Constant3/1 -> Sum/1
  Constant1/1 -> Sum1/2
  Sum1/1 -> Math Function/1
  Sum/1 -> Product/1
  Math Function/1 -> Product/2
  Constant4/1 -> Sum2/1
  Sum2/1 -> Sum3/1  "B"
  Product2/1 -> Sum3/2
  Sum3/1 -> Product1/2
  Constant/1 -> Sum/2, Product4/1
  Product4/1 -> Max = 10 Min=Id_min_abs/1  "min"
  Id_ref (pu)/1 -> Product1/1, MinMax3/1, Product4/2
  MinMax3/1 -> Id_ref_lim/1
  Product3/1 -> Sum2/2
  Product/1 -> Product2/1, Product3/2  "A"
  Constant2/1 -> Sum1/1, Product3/1
  Product1/1 -> MinMax2/1  "Idref_lim"
  MinMax2/1 -> MinMax3/2
  Max = 10 Min=Id_min_abs/1 -> MinMax2/2
  Relational Operator/1 -> Unit Delay/1

== system Controls/Pole 2 Rectifier Control and Protection/Rectifier Controller/Voltage Error ==
  Vd_ref : Inport
  Vd_meas : Inport  Port=2
  Block : Inport  Port=3
  Id_err : Inport  Port=4
  Enable : EnablePort
  Constant1 : Constant  Value=0
  Constant2 : Constant  Value=0
  Constant3 : Constant  Value=Vd_marg
  Constant4 : Constant  Value=Id_marg
  Discrete 1st-Order Filter : powerlib_extras/Discrete  Control Blocks/Discrete 1st-Order Filter  FilterType=Highpass  Tc=0.01  Ts=dt  Initialize=off  Vac_Init=[0.8 -25 60]  Vdc_Init=-0.4  PlotResponse=off  param1=[1 500 0.1]
  MIN:eps MAX:inf : Saturate  UpperLimit=inf  LowerLimit=eps
  Math Function : Math  Operator=reciprocal  SignedPower=on
  Product1 : Product  Inputs=3  InputSameDT=on  SaturateOnIntegerOverflow=on  OutDataTypeStr=Inherit: Same as first input
  S6 : Subsystem  mask(Limiter with External Limits){}
      mask Display: disp('      Limiter\n')
  Sum3 : Sum  Inputs=+--  InputSameDT=on  SaturateOnIntegerOverflow=on  OutDataTypeStr=Inherit: Same as first input
  Switch2 : Switch  Threshold=0.5
  ERR_V : Outport
  wires:
  Sum3/1 -> Switch2/3
  Vd_ref/1 -> Sum3/1
  Vd_meas/1 -> Sum3/2
  Constant1/1 -> Switch2/1
  Block/1 -> Switch2/2
  Switch2/1 -> ERR_V/1  "ERR"
  Constant2/1 -> S6/3(MIN)
  S6/1("  ") -> Product1/3
  Math Function/1 -> Product1/2
  MIN:eps MAX:inf/1 -> Math Function/1
  Constant4/1 -> MIN:eps MAX:inf/1, S6/1(MAX)
  Product1/1 -> Discrete 1st-Order Filter/1
  Discrete 1st-Order Filter/1 -> Sum3/3  "dV"
  Id_err/1 -> S6/2(In)
  Constant3/1 -> Product1/1

== system Controls/Pole 2 Rectifier Control and Protection/Rectifier Controller/Voltage Regulator ==
  Max_i : Inport
  Min_i : Inport  Port=2
  ERR : Inport  Port=3
  Max_pi : Inport  Port=4
  Min_pi : Inport  Port=5
  Alpha_lin : Inport  Port=6
  Max_lin : Inport  Port=7
  Min_lin : Inport  Port=8
  Inv : Inport  Port=9
  Kp : Inport  Port=10
  Ki : Inport  Port=11
  Enable : EnablePort
  Voltage Regulator : Subsystem  mask(PI Regulator  With  External  Limits (Discrete)){Kp=Kp_V, Ki=Ki_V, IC_i=ICi_V, On_lin=on, pas=dt}
      mask prompts: Kp "Kp (deg/pu):"; Ki "Ki (deg/pu/s):"; IC_i "Integrator Initial Condition (deg):"; On_lin "Linearization  (On)"; pas "Sample time (s):"
      mask help: For the linearization it is important to specifie the mode of operation i.e. rectifier or inverter (negation of rectifier).
      mask Display: disp('PI Regulator\nWith external limits\n(Linearized Kp)\n(Discrete)\n\n')
  Alpha_ord : Outport
  wires:
  Kp/1 -> Voltage Regulator/10(Kp)
  Ki/1 -> Voltage Regulator/11(Ki)
  Voltage Regulator/1(Alpha_ord) -> Alpha_ord/1
  Max_i/1 -> Voltage Regulator/1(Max_i)
  Min_i/1 -> Voltage Regulator/2(Min_i)
  ERR/1 -> Voltage Regulator/3(ERR)
  Max_pi/1 -> Voltage Regulator/4(Max_pi)
  Min_pi/1 -> Voltage Regulator/5(Min_pi)
  Alpha_lin/1 -> Voltage Regulator/6(Alpha_lin)
  Max_lin/1 -> Voltage Regulator/7(Max_lin)
  Min_lin/1 -> Voltage Regulator/8(Min_lin)
  Inv/1 -> Voltage Regulator/9(Inv)

== system Controls/Pole 2 Rectifier Control and Protection/Rectifier Controller/alpha_init ==
  In1 : Inport  PortDimensions=1
  IC : InitialCondition  Value=min([ICi_V,ICi_I,ICi_G])
  Out1 : Outport
  wires:
  In1/1 -> IC/1
  IC/1 -> Out1/1

== system Controls/Pole 2 Rectifier Control and Protection/Rectifier Protections/DC Fault Protection (DCPROT) ==
  note: DC Fault Protection (only in Rectifier)
  VdL (pu) : Inport
  Deblocked : Inport  Port=2  OutDataTypeStr=boolean
  Lock : Inport  Port=3
  Enabled Subsystem : Subsystem  TreatAsAtomicUnit=on
  Forced_alpha : Outport
  wires:
  Enabled Subsystem/1(Forced_alpha) -> Forced_alpha/1
  Deblocked/1 -> Enabled Subsystem/2(Deblocked)
  Lock/1 -> Enabled Subsystem/3(Lock)
  VdL (pu)/1 -> Enabled Subsystem/1(VdL (pu))

== system Controls/Pole 2 Rectifier Control and Protection/Rectifier Protections/Informations ==
  note: The DC fault protection (DCPROT) and the Low AC voltage detection (LACVD) constitutes the
      | protectives functions at the rectifier. The DC fault protection detects a fault on the DC line and tries to
      | extinguish the fault current by ordering a Forced alpha operation during a fixed duration.
  note: DESCRIPTION
  note: Silvano Casoria (Hydro-Quebec)
  note: DC Protections - Rectifier
  note: The LACVD detects a low AC voltage condition on the rectifier commutation bus and sends a signal
      | (Lock) to the DCPROT in order to prevent the detection of a DC fault when the drop in the DC voltage is
      | due to a fault on the AC side. The LACVD at the inverter sends also a signal to lock the DCPROT for the
      | same reason.
  note: The  DCPROT detects a fault on the DC line and tries to extinguish the fault current by ordering a Forced
      | alpha operation for a fixed duration.

== system Controls/Pole 2 Rectifier Control and Protection/Rectifier Protections/Low AC Voltage Detection (LACVD) ==
  note: Low AC Voltage Detection
  Uac (pu) : Inport
  Enabled Subsystem : Subsystem  TreatAsAtomicUnit=on
  Low_AC_Voltage : Outport
  wires:
  Enabled Subsystem/1(Low_AC_Voltage) -> Low_AC_Voltage/1
  Uac (pu)/1 -> Enabled Subsystem/1(Uac (pu))

== system Controls/Pole 2 Rectifier Control and Protection/Rectifier Protections/Udio_6p ==
  note: Silvano Casoria
      | Power System Laboratory, IREQ
      | Hydro-Quebec
  note: Three-phase full-wave rectification
  Uabc (pu) : Inport
  MinMax : MinMax  Function=max  InputSameDT=on  SaturateOnIntegerOverflow=on
  MinMax1 : MinMax  InputSameDT=on  SaturateOnIntegerOverflow=on
  Sum : Sum  Inputs=+-  InputSameDT=on  SaturateOnIntegerOverflow=on  OutDataTypeStr=Inherit: Same as first input
  conversion pu ac->dc : Gain  Gain=pi/(3*sqrt(3))  SaturateOnIntegerOverflow=on  OutDataTypeStr=Inherit: Same as input  ParamDataTypeStr=Inherit: Same as input
  Udio_6p : Outport
  wires:
  MinMax1/1 -> Sum/2
  MinMax/1 -> Sum/1
  Uabc (pu)/1 -> MinMax/1, MinMax1/1
  Sum/1 -> conversion pu ac->dc/1
  conversion pu ac->dc/1 -> Udio_6p/1

== system Controls/fault_trigger/faultgen/Subsystem ==
  pertset : Inport
  Tacq : Inport  Port=2
  swth : Inport  Port=3
  Bias : Bias  Bias=-0.5  SaturateOnIntegerOverflow=off
  Data Type Conversion : DataTypeConversion  SaturateOnIntegerOverflow=off  RndMeth=Floor
  Demux4 : Demux  Outputs=2
      settings: DisplayOption=none
  Discrete-Time Integrator1 : DiscreteIntegrator  gainval=2  SampleTime=-1  LimitOutput=on  LowerSaturationLimit=0  ICPrevOutput=DiscIntNeverNeededParam  ICPrevScaledInput=DiscIntNeverNeededParam
  Divide : Product  Inputs=*/
  Gain : Gain  Gain=1/2
  Multiport Switch : MultiPortSwitch  Inputs=2  SaturateOnIntegerOverflow=off  InputSameDT=off
  Product2 : Product  Inputs=3  RndMeth=Zero
  Relational Operator1 : RelationalOperator  OutDataTypeStr=boolean  InputSameDT=off
  Saturation : Saturate  UpperLimit=2  LowerLimit=1
  pertb : Outport
  wires:
  Product2/1 -> pertb/1
  pertset/1 -> Demux4/1
  Tacq/1 -> Gain/1, Divide/2
  swth/1 -> Relational Operator1/2
  Demux4/2 -> Product2/2, Saturation/1
  Demux4/1 -> Product2/1
  Multiport Switch/1 -> Product2/3
  Divide/1 -> Multiport Switch/3  "triangle"
  Saturation/1 -> Multiport Switch/1
  Discrete-Time Integrator1/1 -> Divide/1
  Data Type Conversion/1 -> Multiport Switch/2, Bias/1  "square"
  Bias/1 -> Discrete-Time Integrator1/1
  Relational Operator1/1 -> Data Type Conversion/1
  Gain/1 -> Relational Operator1/1

== system Controls/fault_trigger/faultgen/Tdr ==
  T_p : Inport
  Add : Sum
  Demux : Demux  Outputs=3
  Discrete-Time Integrtor : DiscreteIntegrator  ExternalReset=rising  SampleTime=-1  ICPrevOutput=DiscIntNeverNeededParam  ICPrevScaledInput=DiscIntNeverNeededParam
  Divide : Product  Inputs=*/
  Relational Operator : RelationalOperator  OutDataTypeStr=boolean  InputSameDT=off
  Unit Delay : UnitDelay  SampleTime=Ts  HasFrameUpgradeWarning=on
  t : Outport
  wires:
  Unit Delay/1 -> Relational Operator/1
  Relational Operator/1 -> Discrete-Time Integrtor/2
  Discrete-Time Integrtor/1 -> Add/2, Unit Delay/1
  Divide/1 -> Discrete-Time Integrtor/1
  T_p/1 -> Demux/1
  Demux/1 -> Add/1
  Demux/2 -> Divide/1, Relational Operator/2
  Demux/3 -> Divide/2
  Add/1 -> t/1

== system Controls/fault_trigger/faultgen/Tst ==
  T_p : Inport
  Add : Sum
  Demux : Demux  Outputs=3
  Discrete-Time Integrtor : DiscreteIntegrator  ExternalReset=rising  SampleTime=-1  ICPrevOutput=DiscIntNeverNeededParam  ICPrevScaledInput=DiscIntNeverNeededParam
  Divide : Product  Inputs=*/
  Relational Operator : RelationalOperator  OutDataTypeStr=boolean  InputSameDT=off
  Unit Delay : UnitDelay  SampleTime=Ts  HasFrameUpgradeWarning=on
  t : Outport
  wires:
  Unit Delay/1 -> Relational Operator/1
  Add/1 -> t/1
  Demux/3 -> Divide/2
  Demux/2 -> Relational Operator/2, Divide/1
  Demux/1 -> Add/1
  T_p/1 -> Demux/1
  Divide/1 -> Discrete-Time Integrtor/1
  Discrete-Time Integrtor/1 -> Add/2, Unit Delay/1
  Relational Operator/1 -> Discrete-Time Integrtor/2
